simulink model "PIDsim"  (R2021b)
settings: Solver=VariableStepAuto  StartTime=0.0  StopTime=6  RelTol=1e-3
values from neighbouring files (symbols this model uses):
  d0 = 14    [LQRsetup.m]    (also in PIDsetup.m; datasheet.m = 0.01228; setup.m = 0.01228)
  deltasK = [1 1.24795431189 1.45684423475 1.48717948718 1.74052841115 1.95712837134 1.97435897436 2.24575469341 2.46153846154 2.4683802841 2.75898820638 2.94871794872 ... (115 elements, 1x115)]    [Kvals.mat]
  grad_est = [63.5917222568 53.9084270066 47.7791802541 47.0030992304 41.3884915055 37.5533538094 37.2785627315 33.4260707545 30.8880841006 30.8139012145 27.9615104281 26.3679564487 ... (115 elements, 1x115)]    [Kvals.mat]
  mG = gc(1)    [LQRsetup.m]    (also in PIDsetup.m)
  qG = gc(2)    [LQRsetup.m]    (also in PIDsetup.m)
  start = d0    (= 14)    [LQRsetup.m]    (also in PIDsetup.m = 10.5)
libraries: spsFirstOrderFilterLib x1, MAGLEV_components x1, slpidlib x1
settings Model: Creator=dfigu  LastModifiedBy=dfigu

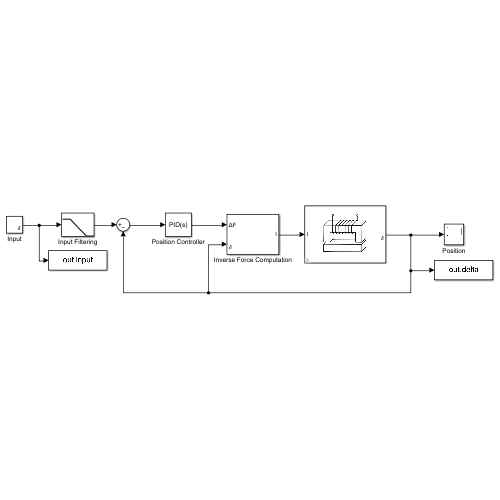
[thumbnail: Simulink's stored preview of the top-level diagram]
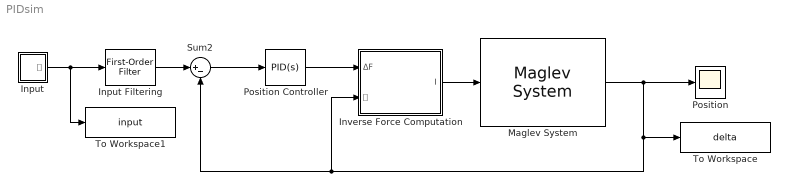
== system PIDsim ==
  Input : Subsystem
  Input Filtering : spsFirstOrderFilterLib/First-Order Filter  FilterType=Lowpass  Tc=0.1  Ts=0  Initialize=on  Vac_Init=[0, 0, 0]  Vdc_Init=d0  PlotResponse=off  FreqRange="[0,  200,  1]"
  Inverse Force Computation : Subsystem
  Maglev System : MAGLEV_components/Maglev System
      link override "Mechanical System/Integrator, Second-Order": ICX=0/1000
  Position : Scope
  Position Controller : slpidlib/PID Controller  Controller=PID  Form=Parallel  TimeDomain=Continuous-time  UseExternalTs=off  SampleTime=-1  IntegratorMethod=Forward Euler  FilterMethod=Forward Euler  ControllerParametersSource=internal  P=-2  I=-20  D=-0.1  UseFilter=on  N=100  TunerSelectOption=Transfer Function Based (PID Tuner App)  InitialConditionSource=internal  InitialConditionForIntegrator=0  InitialConditionForFilter=0  DifferentiatorICPrevScaledInput=0  ExternalReset=none  TrackingMode=off  Kt=1  LimitOutput=off  SatLimitsSource=internal  UpperSaturationLimit=inf  LowerSaturationLimit=-inf  LinearizeAsGain=on  AntiWindupMode=none  Kb=1  POutMin=[]  POutMax=[]  IOutMin=[]  IOutMax=[]  DOutMin=[]  DOutMax=[]  NOutMin=[]  NOutMax=[]  SumOutMin=[]  SumOutMax=[]  SaturationOutMin=[]  SaturationOutMax=[]  PParamMin=[]  PParamMax=[]  IParamMin=[]  IParamMax=[]  DParamMin=[]  DParamMax=[]  NParamMin=[]  NParamMax=[]  KbParamMin=[]  KbParamMax=[]  KtParamMin=[]  KtParamMax=[]  KbOutMin=[]  KbOutMax=[]  KtOutMin=[]  KtOutMax=[]  IntegratorOutMin=[]  IntegratorOutMax=[]  FilterOutMin=[]  FilterOutMax=[]  SumI1OutMin=[]  SumI1OutMax=[]  SumI2OutMin=[]  SumI2OutMax=[]  SumI3OutMin=[]  SumI3OutMax=[]  SumI4OutMin=[]  SumI4OutMax=[]  SumDOutMin=[]  SumDOutMax=[]  DifferentiatorOutMin=[]  DifferentiatorOutMax=[]  FilterDiffOutCoefMin=[]  FilterDiffOutCoefMax=[]  ReciprocalOutMin=[]  ReciprocalOutMax=[]  SumDenOutMin=[]  SumDenOutMax=[]  SumNumOutMin=[]  SumNumOutMax=[]  DivideOutMin=[]  DivideOutMax=[]  UdiffTsProdOutMin=[]  UdiffTsProdOutMax=[]  NTsProdOutMin=[]  NTsProdOutMax=[]  UintegralTsProdOutMin=[]  UintegralTsProdOutMax=[]  UngainTsProdOutMin=[]  UngainTsProdOutMax=[]  IntegratorContinuousStateAttributes=''  IntegratorStateMustResolveToSignalObject=off  IntegratorRTWStateStorageClass=Auto  FilterContinuousStateAttributes=''  FilterStateMustResolveToSignalObject=off  FilterRTWStateStorageClass=Auto  ParallelPVariant=InternalParameters  IdealPVariant=Disabled  IVariant=InternalParameters  DVariant=InternalParameters  IntegratorVariant=Continuous  SatVariant=Disabled  AWVariant=Passthrough  PCopyVariant=Disabled  TRVariant=Disabled  FdbkBlocksVariant=Forward  IdealPFdbkVariant=Disabled  SatFdbkVariant=Disabled  DerivativeFilterVariant=ContFilter  NVariant=InternalParameters  NCopyVariant=Disabled  FilterICVariant=InternalICsFilter  IntegratorICVariant=InternalICs  ExternalResetVariant=Disabled  TRSumVariant=Passthrough  SumFdbkVariant=Disabled  SumVariant=Sum_PID  TsampFilterVariant=InternalTs  TsampNgainVariant=Passthrough  TsampIntegralVariant=Passthrough  ExternalSaturationOutDataTypeStr=Inherit: Same as second input
  Sum2 : Sum  Inputs=|+-
  To Workspace : ToWorkspace  VariableName=delta  SaveFormat=Timeseries  SampleTime=-1
  To Workspace1 : ToWorkspace  VariableName=input  SaveFormat=Timeseries  SampleTime=-1
  wires:
  Maglev System/1 -> Position/1, To Workspace/1, Sum2/2, Inverse Force Computation/2(𝛿)
  Sum2/1 -> Position Controller/1
  Input Filtering/1 -> Sum2/1
  Input/1(𝛿) -> To Workspace1/1, Input Filtering/1
  Position Controller/1 -> Inverse Force Computation/1(ΔF)
  Inverse Force Computation/1(I) -> Maglev System/1

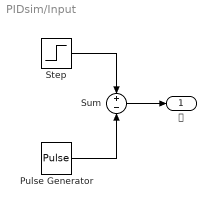
== system PIDsim/Input ==
  Pulse Generator : DiscretePulseGenerator  PulseType=Time based  Amplitude=d0/2  Period=5  PulseWidth=50  PhaseDelay=0.5
  Step : Step  Time=0  Before=d0  After=start  SampleTime=0
  Sum : Sum  Inputs=+|-
  𝛿 : Outport
  wires:
  Sum/1 -> 𝛿/1
  Step/1 -> Sum/1
  Pulse Generator/1 -> Sum/2

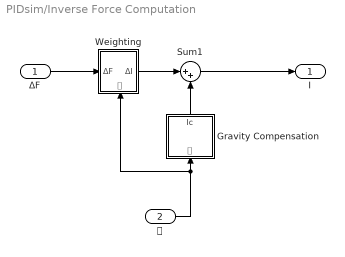
== system PIDsim/Inverse Force Computation ==
  ΔF : Inport
  𝛿 : Inport  Port=2
  Gravity Compensation : Subsystem
  Sum1 : Sum  Inputs=|++
  Weighting : Subsystem
      settings: PortSchema="{\"entries\":[{\"content\":{\"sides\":[{\"content\":{\"connectorIds\":[\"In1\"]},\"type\":\"ConnectorPlacement.EquallySpacedRectSide\",\"uuid\":\"6b47628a-cc08-4372-88a9-27295bde16d5\"},{\"content\":{\"connectorIds\":[\"Out1\"],\"side\":\"RIGHT\"},\"type\":\"ConnectorPlacement.EquallySpacedRectSide\",\"uuid\":\"4e2a4537-6a79-4c56-b693-16bea0361472\"},{\"content\":{\"connectorIds\":[],\"side\":\"TOP\"},\"type\":\"ConnectorPlacement.EquallySpacedRectSide\",\"uuid\":\"9b78d512-7b83-4f33-9e4b-8e81982b1424\"},{\"content\":{\"connectorIds\":[\"In2\"],\"side\":\"BOTTOM\"},\"type\":\"ConnectorPlacement.EquallySpacedRectSide\",\"uuid\":\"7a9ea1e1-3d9a-431d-b0e2-3790018f7e3d\"}]},\"type\":\"ConnectorPlacement.EquallySpacedConnector\",\"uuid\":\"7c66cfeb-15cf-43a6-b9f1-afb80f0c41eb\"}],\"packageUris\":[\"http://schema.mathworks.com/mf0/Connector/R2020b\"],\"version\":\"1.0\"}"
  I : Outport
  wires:
  ΔF/1 -> Weighting/1(ΔF)
  Weighting/1(ΔI) -> Sum1/1
  𝛿/1 -> Weighting/2(𝛿), Gravity Compensation/1(𝛿)
  Gravity Compensation/1(Ic) -> Sum1/2
  Sum1/1 -> I/1

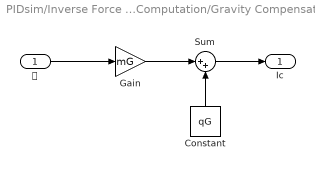
== system PIDsim/Inverse Force Computation/Gravity Compensation ==
  𝛿 : Inport
  Constant : Constant  Value=qG
  Gain : Gain  Gain=mG
  Sum : Sum  Inputs=|++
  Ic : Outport
  wires:
  Gain/1 -> Sum/1
  Sum/1 -> Ic/1
  Constant/1 -> Sum/2
  𝛿/1 -> Gain/1

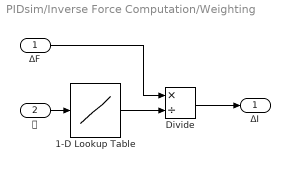
== system PIDsim/Inverse Force Computation/Weighting ==
  ΔF : Inport
  𝛿 : Inport  Port=2
  1-D Lookup Table : Lookup_n-D  NumberOfTableDimensions=1  BreakpointsForDimension1=deltasK  Table=grad_est  InternalRulePriority=Speed  RndMeth=Simplest  InputSameDT=on
  Divide : Product  Inputs=*/
  ΔI : Outport
  wires:
  Divide/1 -> ΔI/1
  1-D Lookup Table/1 -> Divide/2
  ΔF/1 -> Divide/1
  𝛿/1 -> 1-D Lookup Table/1
